simulink model "VIPLStEnCtrl"  (R2018b)
settings: Solver=FixedStepDiscrete  StartTime=0.0  StopTime=10.0  FixedStep=0.01  RelTol=1e-3
undefined symbols (not defined in the file or in its folder): data, DrvStFtEn_Clear, DrvStFtEn_Set, SecRwLtStBkReclnEn_Clear, SecRwLtStBkReclnEn_Set, SecRwLtStFwdBkwdEn_Clear, SecRwLtStFwdBkwdEn_Set, SecRwLtStLgrstUpwdDnwdEn_Clear, SecRwLtStLgrstUpwdDnwdEn_Set, SecRwLtStLtwdRtwdEn_Clear, SecRwLtStLtwdRtwdEn_Set, ThdRwLtStBkReclnEn_Clear, ThdRwLtStBkReclnEn_Set, ThdRwLtStFwdBkwdEn_Clear, ThdRwLtStFwdBkwdEn_Set
libraries: simulink x1
settings Model: Creator=sn2xws  LastModifiedBy=sn2xws
settings DataIOCC: SaveFormat=StructureWithTime
settings OptimizationCC: DefaultParameterBehavior=Inlined  EnhancedBackFolding=on  PassReuseOutputArgsAs=Individual arguments  ZeroExternalMemoryAtStartup=off  ZeroInternalMemoryAtStartup=off  OptimizeBlockOrder=speed  DifferentSizesBufferReuse=on  OptimizationCustomize=off
settings DebuggingCC: ParameterTunabilityLossMsg=error
settings ModelReferenceCC: ModelReferenceNumInstancesAllowed=Single
settings SFSimCC: MATLABDynamicMemAlloc=off
settings RTWCC: SystemTargetFile=autosar.tlc  GenCodeOnly=on  TemplateMakefile=ert_default_tmf  Description=AUTOSAR  GenerateReport=on  IncludeHyperlinkInReport=on  LaunchReport=on  GenerateTraceInfo=on  GenerateTraceReport=on  GenerateTraceReportSl=on  GenerateTraceReportSf=on  GenerateTraceReportEml=on  GenerateCodeMetricsReport=on
settings CodeAppCC: ForceParamTrailComments=on  IgnoreCustomStorageClasses=off  OperatorAnnotations=on  SimulinkDataObjDesc=on  SFDataObjDesc=on  InsertBlockDesc=on
settings STFCustomTargetCC: TargetLangStandard=C99 (ISO)  MultiwordLength=256  ParMdlRefBuildCompliant=on  CompOptLevelCompliant=on  IncludeMdlTerminateFcn=off  CombineOutputUpdateFcns=on  SuppressErrorStatus=on  ERTCustomFileBanners=on  SupportNonFinite=off  SupportComplex=off  SupportContinuousTime=off  SupportNonInlinedSFcns=off  RemoveResetFunc=on  MATLABClassNameForMDSCustomization=Simulink.SoftwareTarget.ERTCustomization  AutosarCompliant=on  UseToolchainInfoCompliant=on  LookupTableObjectStructAxisOrder=2,1,3,4,...  LUTObjectStructOrderEvenSpacing=Size,Table,Breakpoints  SystemTargetFile=autosar.tlc
settings ERTTargetCC: TargetLangStandard=C99 (ISO)  ConcurrentExecutionCompliant=off  IncludeMdlTerminateFcn=off  SuppressErrorStatus=on  SupportNonFinite=off  SupportComplex=off  ModelStepFunctionPrototypeControlCompliant=off  CPPClassGenCompliant=off  AutosarCompliant=on  LookupTableObjectStructAxisOrder=2,1,3,4,...  LUTObjectStructOrderEvenSpacing=Size,Table,Breakpoints  InlinedParameterPlacement=NonHierarchical  ERTCustomFileTemplate=example_file_process.tlc  ERTFilePackagingFormat=Compact

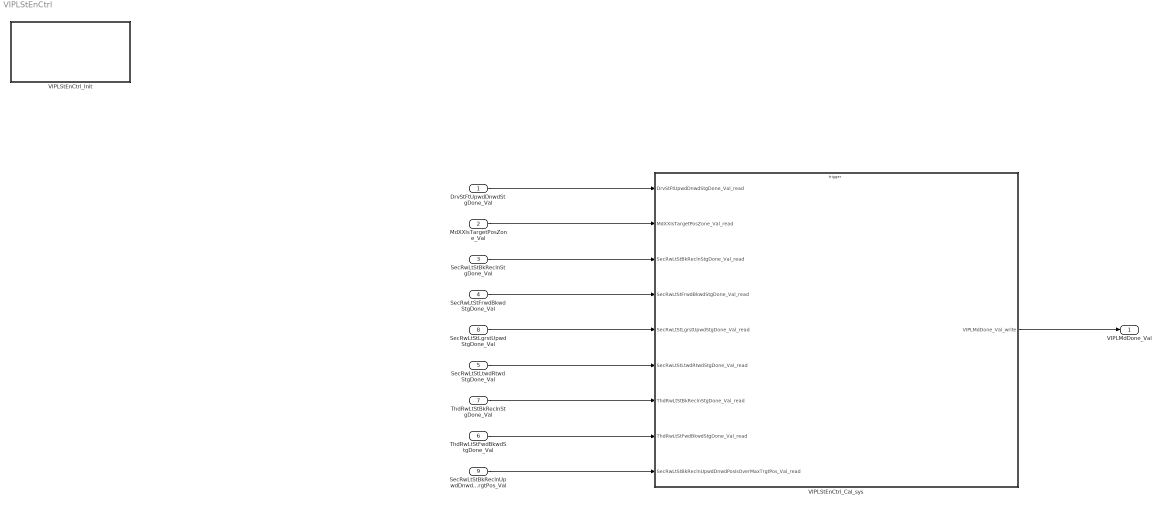
== system VIPLStEnCtrl ==
  DrvStFtUpwdDnwdStgDone_Val : Inport  OutDataTypeStr=boolean  PortDimensions=1
  MdXXIsTargetPosZone_Val : Inport  Port=2  OutDataTypeStr=uint32  PortDimensions=1
  SecRwLtStBkReclnStgDone_Val : Inport  Port=3  OutDataTypeStr=boolean  PortDimensions=1
  SecRwLtStFrwdBkwdStgDone_Val : Inport  Port=4  OutDataTypeStr=boolean  PortDimensions=1
  SecRwLtStLtwdRtwdStgDone_Val : Inport  Port=5  OutDataTypeStr=boolean  PortDimensions=1
  ThdRwLtStFwdBkwdStgDone_Val : Inport  Port=6  OutDataTypeStr=boolean  PortDimensions=1
  ThdRwLtStBkReclnStgDone_Val : Inport  Port=7  OutDataTypeStr=boolean  PortDimensions=1
  SecRwLtStLgrstUpwdStgDone_Val : Inport  Port=8  OutDataTypeStr=boolean  PortDimensions=1
  SecRwLtStBkReclnUpwdDnwdPosIsOverMaxTrgtPos_Val : Inport  Port=9  OutDataTypeStr=boolean  PortDimensions=1
  VIPLStEnCtrl_Cal_sys : Subsystem
  VIPLStEnCtrl_Init : Subsystem
  VIPLMdDone_Val : Outport  OutDataTypeStr=uint8  PortDimensions=1
  wires:
  ThdRwLtStFwdBkwdStgDone_Val/1 -> VIPLStEnCtrl_Cal_sys/8(ThdRwLtStFwdBkwdStgDone_Val_read)
  VIPLStEnCtrl_Cal_sys/1(VIPLMdDone_Val_write) -> VIPLMdDone_Val/1
  DrvStFtUpwdDnwdStgDone_Val/1 -> VIPLStEnCtrl_Cal_sys/1(DrvStFtUpwdDnwdStgDone_Val_read)
  MdXXIsTargetPosZone_Val/1 -> VIPLStEnCtrl_Cal_sys/2(MdXXIsTargetPosZone_Val_read)
  SecRwLtStBkReclnStgDone_Val/1 -> VIPLStEnCtrl_Cal_sys/3(SecRwLtStBkReclnStgDone_Val_read)
  SecRwLtStFrwdBkwdStgDone_Val/1 -> VIPLStEnCtrl_Cal_sys/4(SecRwLtStFrwdBkwdStgDone_Val_read)
  SecRwLtStLgrstUpwdStgDone_Val/1 -> VIPLStEnCtrl_Cal_sys/5(SecRwLtStLgrstUpwdStgDone_Val_read)
  SecRwLtStLtwdRtwdStgDone_Val/1 -> VIPLStEnCtrl_Cal_sys/6(SecRwLtStLtwdRtwdStgDone_Val_read)
  ThdRwLtStBkReclnStgDone_Val/1 -> VIPLStEnCtrl_Cal_sys/7(ThdRwLtStBkReclnStgDone_Val_read)
  SecRwLtStBkReclnUpwdDnwdPosIsOverMaxTrgtPos_Val/1 -> VIPLStEnCtrl_Cal_sys/9(SecRwLtStBkReclnUpwdDnwdPosIsOverMaxTrgtPos_Val_read)

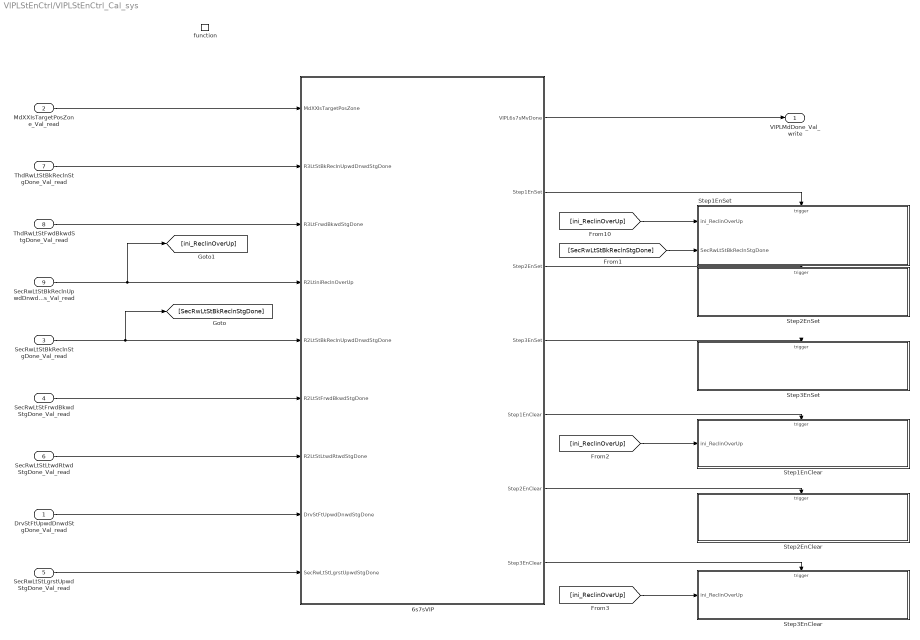
== system VIPLStEnCtrl/VIPLStEnCtrl_Cal_sys ==
  DrvStFtUpwdDnwdStgDone_Val_read : Inport
  MdXXIsTargetPosZone_Val_read : Inport  Port=2
  SecRwLtStBkReclnStgDone_Val_read : Inport  Port=3
  SecRwLtStFrwdBkwdStgDone_Val_read : Inport  Port=4
  SecRwLtStLgrstUpwdStgDone_Val_read : Inport  Port=5
  SecRwLtStLtwdRtwdStgDone_Val_read : Inport  Port=6
  ThdRwLtStBkReclnStgDone_Val_read : Inport  Port=7
  ThdRwLtStFwdBkwdStgDone_Val_read : Inport  Port=8
  SecRwLtStBkReclnUpwdDnwdPosIsOverMaxTrgtPos_Val_read : Inport  Port=9
  function : TriggerPort  TriggerType=function-call  IsSimulinkFunction=on  FunctionName=VIPLStEnCtrl_Cal  VariantControl=(inherit)
  6s7sVIP : Subsystem
  Step1EnClear : Subsystem  TreatAsAtomicUnit=on
  Step1EnSet : Subsystem  TreatAsAtomicUnit=on
  Step2EnClear : Subsystem  TreatAsAtomicUnit=on
  Step2EnSet : Subsystem  TreatAsAtomicUnit=on
  Step3EnClear : Subsystem  TreatAsAtomicUnit=on
  Step3EnSet : Subsystem  TreatAsAtomicUnit=on
  VIPLMdDone_Val_write : Outport
      settings: EnsureOutportIsVirtual=on
  wires:
  6s7sVIP/1(VIPL6s7sMvDone) -> VIPLMdDone_Val_write/1
  MdXXIsTargetPosZone_Val_read/1 -> 6s7sVIP/1(MdXXIsTargetPosZone)
  ThdRwLtStBkReclnStgDone_Val_read/1 -> 6s7sVIP/2(R3LtStBkReclnUpwdDnwdStgDone)
  ThdRwLtStFwdBkwdStgDone_Val_read/1 -> 6s7sVIP/3(R3LtFrwdBkwdStgDone)
  SecRwLtStBkReclnStgDone_Val_read/1 -> [SecRwLtStBkReclnStgDone], 6s7sVIP/5(R2LtStBkReclnUpwdDnwdStgDone)
  SecRwLtStFrwdBkwdStgDone_Val_read/1 -> 6s7sVIP/6(R2LtStFrwdBkwdStgDone)
  SecRwLtStLtwdRtwdStgDone_Val_read/1 -> 6s7sVIP/7(R2LtStLtwdRtwdStgDone)
  SecRwLtStLgrstUpwdStgDone_Val_read/1 -> 6s7sVIP/9(SecRwLtStLgrstUpwdStgDone)
  DrvStFtUpwdDnwdStgDone_Val_read/1 -> 6s7sVIP/8(DrvStFtUpwdDnwdStgDone)
  [ini_ReclinOverUp] -> Step1EnSet/1(ini_ReclinOverUp)
  6s7sVIP/6(Step2EnClear) -> Step2EnClear/Trigger
  6s7sVIP/7(Step3EnClear) -> Step3EnClear/Trigger
  6s7sVIP/4(Step3EnSet) -> Step3EnSet/Trigger
  [SecRwLtStBkReclnStgDone] -> Step1EnSet/2(SecRwLtStBkReclnStgDone)
  6s7sVIP/3(Step2EnSet) -> Step2EnSet/Trigger
  6s7sVIP/2(Step1EnSet) -> Step1EnSet/Trigger
  6s7sVIP/5(Step1EnClear) -> Step1EnClear/Trigger
  [ini_ReclinOverUp] -> Step1EnClear/1(ini_ReclinOverUp)
  [ini_ReclinOverUp] -> Step3EnClear/1(ini_ReclinOverUp)
  SecRwLtStBkReclnUpwdDnwdPosIsOverMaxTrgtPos_Val_read/1 -> [ini_ReclinOverUp], 6s7sVIP/4(R2LtiniReclnOverUp)

== system VIPLStEnCtrl/VIPLStEnCtrl_Init ==
  Event Listener : EventListener  EventName=reset

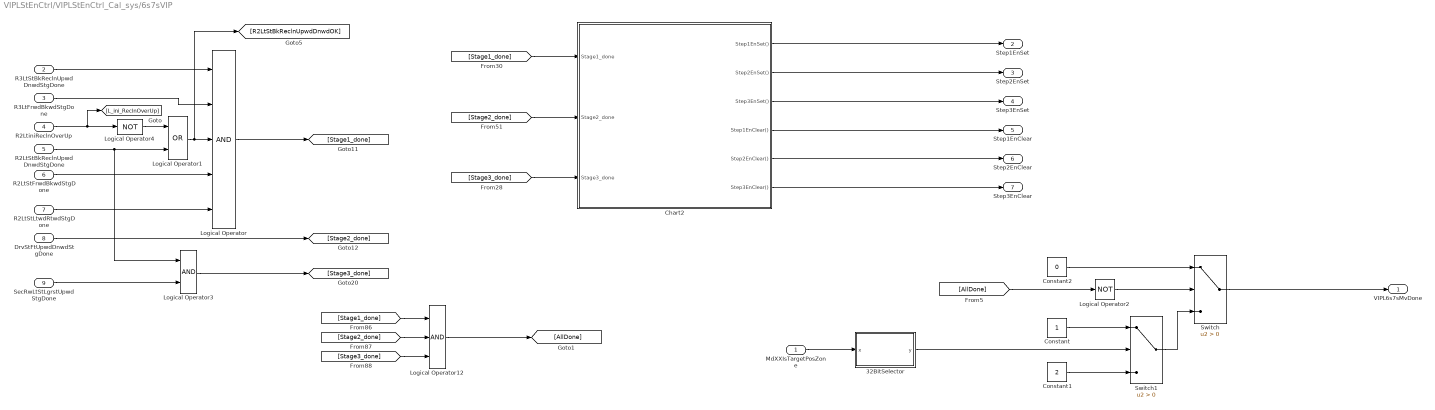
== system VIPLStEnCtrl/VIPLStEnCtrl_Cal_sys/6s7sVIP ==
  MdXXIsTargetPosZone : Inport
  R3LtStBkReclnUpwdDnwdStgDone : Inport  Port=2
  R3LtFrwdBkwdStgDone : Inport  Port=3
  R2LtiniReclnOverUp : Inport  Port=4
  R2LtStBkReclnUpwdDnwdStgDone : Inport  Port=5
  R2LtStFrwdBkwdStgDone : Inport  Port=6
  R2LtStLtwdRtwdStgDone : Inport  Port=7
  DrvStFtUpwdDnwdStgDone : Inport  Port=8
  SecRwLtStLgrstUpwdStgDone : Inport  Port=9
  32BitSelector : Subsystem  mask(32 Bit Selector){BitNum=9}
      mask prompts: BitNum "Select Bit Number"
      mask help: Allows selection of a particular bit (0-31) out of a packed word up to 32 bits long. Output will be true if the bit number selected via the mask parameter is equal to one.
      mask TypeOptions BitNum: 0 | 1 | 2 | 3 | 4 | 5 | 6 | 7 | 8 | 9 | 10 | 11 | 12 | 13 | 14 | 15 | 16 | 17 | 18 | 19 | 20 | 21 | 22 | 23 | 24 | 25 | 26 | 27 | 28 | 29 | 30 | 31
      mask Display:
      | text(0.5, 0.8,'BIT','horizontalAlignment','center')
      | text(0.5, 0.5,'SELECTOR','horizontalAlignment','center')
      | text(0.5, 0.2,['-- Bit ',char(get_param(gcb,'BitNum')),' --'],'horizontalAlignment','center')
  Chart2 : Stateflow chart  TreatAsAtomicUnit=on
  Constant : Constant  OutDataTypeStr=uint8
  Constant1 : Constant  Value=2  OutDataTypeStr=uint8
  Constant2 : Constant  Value=0  OutDataTypeStr=uint8
  Logical Operator : Logic  Inputs=5  AllPortsSameDT=off  OutDataTypeStr=boolean
  Logical Operator1 : Logic  Operator=OR  AllPortsSameDT=off  OutDataTypeStr=boolean
  Logical Operator12 : Logic  Inputs=3  AllPortsSameDT=off  OutDataTypeStr=boolean
  Logical Operator2 : Logic  Operator=NOT  AllPortsSameDT=off  OutDataTypeStr=boolean
  Logical Operator3 : Logic  AllPortsSameDT=off  OutDataTypeStr=boolean
  Logical Operator4 : Logic  Operator=NOT  AllPortsSameDT=off  OutDataTypeStr=boolean
  Switch : Switch  Criteria=u2 > Threshold
  Switch1 : Switch  Criteria=u2 > Threshold
  VIPL6s7sMvDone : Outport
  Step1EnSet : Outport  Port=2
  Step2EnSet : Outport  Port=3
  Step3EnSet : Outport  Port=4
  Step1EnClear : Outport  Port=5
  Step2EnClear : Outport  Port=6
  Step3EnClear : Outport  Port=7
  wires:
  [Stage1_done] -> Chart2/1(Stage1_done)
  SecRwLtStLgrstUpwdStgDone/1 -> Logical Operator3/2
  Logical Operator4/1 -> Logical Operator1/1
  [Stage3_done] -> Logical Operator12/3
  R3LtFrwdBkwdStgDone/1 -> Logical Operator/2
  [Stage2_done] -> Chart2/2(Stage2_done)
  R2LtStBkReclnUpwdDnwdStgDone/1 -> Logical Operator1/2, Logical Operator3/1
  Logical Operator1/1 -> [R2LtStBkReclnUpwdDnwdOK], Logical Operator/3
  Logical Operator/1 -> [Stage1_done]
  R3LtStBkReclnUpwdDnwdStgDone/1 -> Logical Operator/1
  Logical Operator3/1 -> [Stage3_done]
  R2LtiniReclnOverUp/1 -> [L_ini_ReclnOverUp], Logical Operator4/1
  R2LtStFrwdBkwdStgDone/1 -> Logical Operator/4
  DrvStFtUpwdDnwdStgDone/1 -> [Stage2_done]
  MdXXIsTargetPosZone/1 -> 32BitSelector/1(x)
  Logical Operator12/1 -> [AllDone]
  [Stage2_done] -> Logical Operator12/2
  R2LtStLtwdRtwdStgDone/1 -> Logical Operator/5
  [Stage1_done] -> Logical Operator12/1
  [Stage3_done] -> Chart2/3(Stage3_done)
  Chart2/1(Step1EnSet()) -> Step1EnSet/1
  Chart2/2(Step2EnSet()) -> Step2EnSet/1
  Chart2/3(Step3EnSet()) -> Step3EnSet/1
  Chart2/4(Step1EnClear()) -> Step1EnClear/1
  Chart2/5(Step2EnClear()) -> Step2EnClear/1
  Chart2/6(Step3EnClear()) -> Step3EnClear/1
  Switch1/1 -> Switch/3
  Switch/1 -> VIPL6s7sMvDone/1
  Constant2/1 -> Switch/1
  Constant1/1 -> Switch1/3
  Constant/1 -> Switch1/1
  Logical Operator2/1 -> Switch/2
  [AllDone] -> Logical Operator2/1
  32BitSelector/1(y) -> Switch1/2

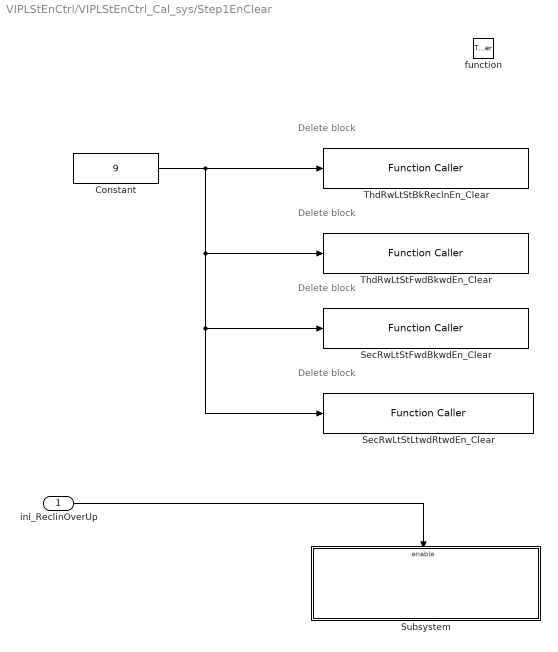
== system VIPLStEnCtrl/VIPLStEnCtrl_Cal_sys/Step1EnClear ==
  note: Delete block
  note: Delete block
  note: Delete block
  note: Delete block
  ini_ReclinOverUp : Inport
  function : TriggerPort  TriggerType=function-call  VariantControl=Variant
  Constant : Constant  Value=9  OutDataTypeStr=uint8
  SecRwLtStFwdBkwdEn_Clear : FunctionCaller  FunctionPrototype=SecRwLtStFwdBkwdEn_Clear(data)  InputArgumentSpecifications=uint8(1)
  SecRwLtStLtwdRtwdEn_Clear : FunctionCaller  FunctionPrototype=SecRwLtStLtwdRtwdEn_Clear(data)  InputArgumentSpecifications=uint8(1)
  Subsystem : Subsystem
  ThdRwLtStBkReclnEn_Clear : FunctionCaller  FunctionPrototype=ThdRwLtStBkReclnEn_Clear(data)  InputArgumentSpecifications=uint8(1)
  ThdRwLtStFwdBkwdEn_Clear : FunctionCaller  FunctionPrototype=ThdRwLtStFwdBkwdEn_Clear(data)  InputArgumentSpecifications=uint8(1)
  wires:
  Constant/1 -> ThdRwLtStBkReclnEn_Clear/1, SecRwLtStFwdBkwdEn_Clear/1, SecRwLtStLtwdRtwdEn_Clear/1, ThdRwLtStFwdBkwdEn_Clear/1
  ini_ReclinOverUp/1 -> Subsystem/Enable

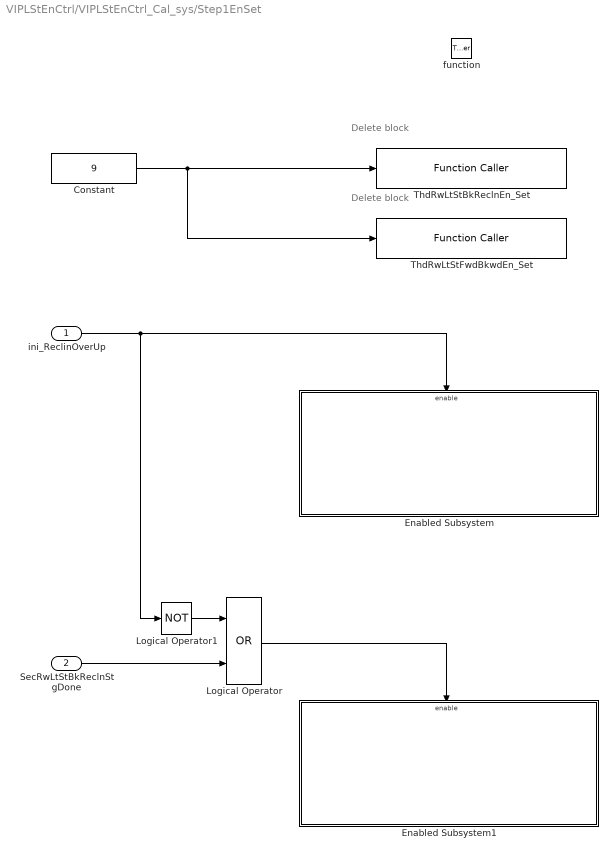
== system VIPLStEnCtrl/VIPLStEnCtrl_Cal_sys/Step1EnSet ==
  note: Delete block
  note: Delete block
  ini_ReclinOverUp : Inport
  SecRwLtStBkReclnStgDone : Inport  Port=2
  function : TriggerPort  TriggerType=function-call  VariantControl=Variant
  Constant : Constant  Value=9  OutDataTypeStr=uint8
  Enabled Subsystem : Subsystem  TreatAsAtomicUnit=on
  Enabled Subsystem1 : Subsystem  TreatAsAtomicUnit=on
  Logical Operator : Logic  Operator=OR  AllPortsSameDT=off  OutDataTypeStr=boolean
  Logical Operator1 : Logic  Operator=NOT  AllPortsSameDT=off  OutDataTypeStr=boolean
  ThdRwLtStBkReclnEn_Set : FunctionCaller  FunctionPrototype=ThdRwLtStBkReclnEn_Set(data)  InputArgumentSpecifications=uint8(1)
  ThdRwLtStFwdBkwdEn_Set : FunctionCaller  FunctionPrototype=ThdRwLtStFwdBkwdEn_Set(data)  InputArgumentSpecifications=uint8(1)
  wires:
  Constant/1 -> ThdRwLtStBkReclnEn_Set/1, ThdRwLtStFwdBkwdEn_Set/1
  ini_ReclinOverUp/1 -> Logical Operator1/1, Enabled Subsystem/Enable
  SecRwLtStBkReclnStgDone/1 -> Logical Operator/2
  Logical Operator1/1 -> Logical Operator/1
  Logical Operator/1 -> Enabled Subsystem1/Enable

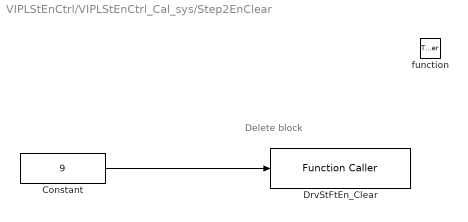
== system VIPLStEnCtrl/VIPLStEnCtrl_Cal_sys/Step2EnClear ==
  note: Delete block
  function : TriggerPort  TriggerType=function-call  VariantControl=Variant
  Constant : Constant  Value=9  OutDataTypeStr=uint8
  DrvStFtEn_Clear : FunctionCaller  FunctionPrototype=DrvStFtEn_Clear(data)  InputArgumentSpecifications=uint8(1)
  wires:
  Constant/1 -> DrvStFtEn_Clear/1

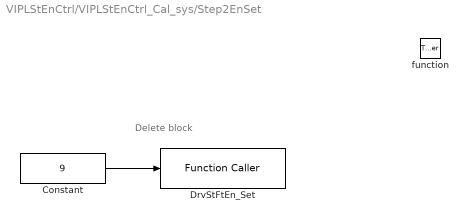
== system VIPLStEnCtrl/VIPLStEnCtrl_Cal_sys/Step2EnSet ==
  note: Delete block
  function : TriggerPort  TriggerType=function-call  VariantControl=Variant
  Constant : Constant  Value=9  OutDataTypeStr=uint8
  DrvStFtEn_Set : FunctionCaller  FunctionPrototype=DrvStFtEn_Set(data)  InputArgumentSpecifications=uint8(1)
  wires:
  Constant/1 -> DrvStFtEn_Set/1

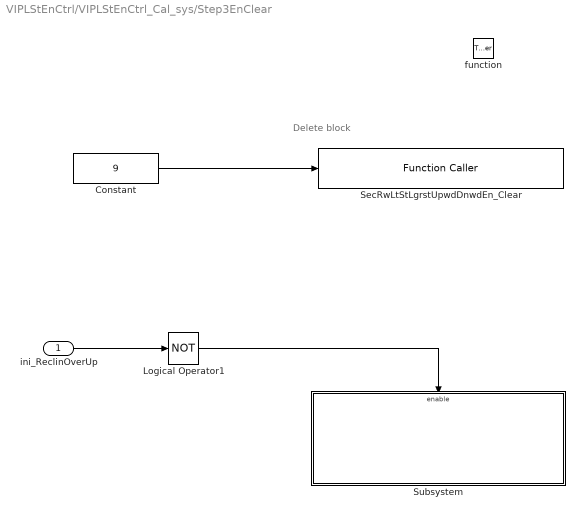
== system VIPLStEnCtrl/VIPLStEnCtrl_Cal_sys/Step3EnClear ==
  note: Delete block
  ini_ReclinOverUp : Inport
  function : TriggerPort  TriggerType=function-call  VariantControl=Variant
  Constant : Constant  Value=9  OutDataTypeStr=uint8
  Logical Operator1 : Logic  Operator=NOT  AllPortsSameDT=off  OutDataTypeStr=boolean
  SecRwLtStLgrstUpwdDnwdEn_Clear : FunctionCaller  FunctionPrototype=SecRwLtStLgrstUpwdDnwdEn_Clear(data)  InputArgumentSpecifications=uint8(1)
  Subsystem : Subsystem
  wires:
  Constant/1 -> SecRwLtStLgrstUpwdDnwdEn_Clear/1
  ini_ReclinOverUp/1 -> Logical Operator1/1
  Logical Operator1/1 -> Subsystem/Enable

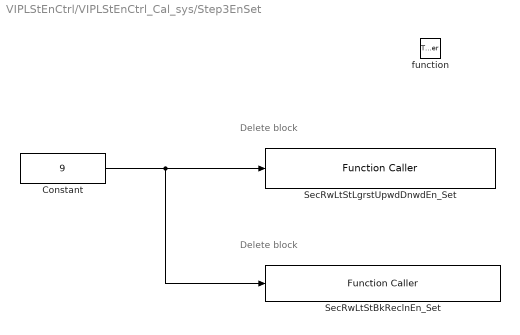
== system VIPLStEnCtrl/VIPLStEnCtrl_Cal_sys/Step3EnSet ==
  note: Delete block
  note: Delete block
  function : TriggerPort  TriggerType=function-call  VariantControl=Variant
  Constant : Constant  Value=9  OutDataTypeStr=uint8
  SecRwLtStBkReclnEn_Set : FunctionCaller  FunctionPrototype=SecRwLtStBkReclnEn_Set(data)  InputArgumentSpecifications=uint8(1)
  SecRwLtStLgrstUpwdDnwdEn_Set : FunctionCaller  FunctionPrototype=SecRwLtStLgrstUpwdDnwdEn_Set(data)  InputArgumentSpecifications=uint8(1)
  wires:
  Constant/1 -> SecRwLtStBkReclnEn_Set/1, SecRwLtStLgrstUpwdDnwdEn_Set/1

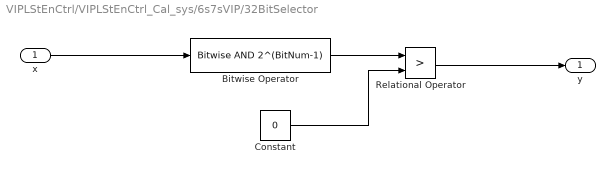
== system VIPLStEnCtrl/VIPLStEnCtrl_Cal_sys/6s7sVIP/32BitSelector ==
  x : Inport
  Bitwise Operator : simulink/Logic and Bit Operations/Bitwise Operator  logicop=AND  UseBitMask=on  BitMask=2^(BitNum-1)  BitMaskRealWorld=Stored Integer
  Constant : Constant  Value=0  OutDataTypeStr=uint32
  Relational Operator : RelationalOperator  Operator=>  OutDataTypeStr=boolean  RndMeth=Simplest
  y : Outport
  wires:
  Relational Operator/1 -> y/1
  Constant/1 -> Relational Operator/2
  x/1 -> Bitwise Operator/1
  Bitwise Operator/1 -> Relational Operator/1

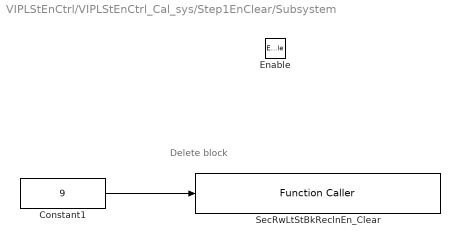
== system VIPLStEnCtrl/VIPLStEnCtrl_Cal_sys/Step1EnClear/Subsystem ==
  note: Delete block
  Enable : EnablePort
  Constant1 : Constant  Value=9  OutDataTypeStr=uint8
  SecRwLtStBkReclnEn_Clear : FunctionCaller  FunctionPrototype=SecRwLtStBkReclnEn_Clear(data)  InputArgumentSpecifications=uint8(1)
  wires:
  Constant1/1 -> SecRwLtStBkReclnEn_Clear/1

== system VIPLStEnCtrl/VIPLStEnCtrl_Cal_sys/Step1EnSet/Enabled Subsystem ==
  note: Delete block
  Enable : EnablePort
  Constant : Constant  Value=9  OutDataTypeStr=uint8
  SecRwLtStBkReclnEn_Set : FunctionCaller  FunctionPrototype=SecRwLtStBkReclnEn_Set(data)  InputArgumentSpecifications=uint8(1)
  wires:
  Constant/1 -> SecRwLtStBkReclnEn_Set/1

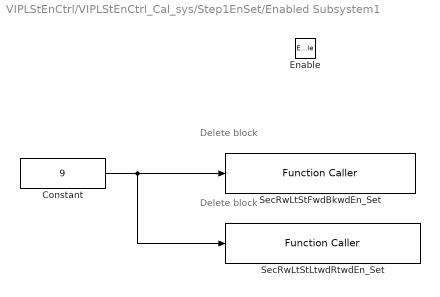
== system VIPLStEnCtrl/VIPLStEnCtrl_Cal_sys/Step1EnSet/Enabled Subsystem1 ==
  note: Delete block
  note: Delete block
  Enable : EnablePort
  Constant : Constant  Value=9  OutDataTypeStr=uint8
  SecRwLtStFwdBkwdEn_Set : FunctionCaller  FunctionPrototype=SecRwLtStFwdBkwdEn_Set(data)  InputArgumentSpecifications=uint8(1)
  SecRwLtStLtwdRtwdEn_Set : FunctionCaller  FunctionPrototype=SecRwLtStLtwdRtwdEn_Set(data)  InputArgumentSpecifications=uint8(1)
  wires:
  Constant/1 -> SecRwLtStFwdBkwdEn_Set/1, SecRwLtStLtwdRtwdEn_Set/1

== system VIPLStEnCtrl/VIPLStEnCtrl_Cal_sys/Step3EnClear/Subsystem ==
  note: Delete block
  Enable : EnablePort
  Constant1 : Constant  Value=9  OutDataTypeStr=uint8
  SecRwLtStBkReclnEn_Clear : FunctionCaller  FunctionPrototype=SecRwLtStBkReclnEn_Clear(data)  InputArgumentSpecifications=uint8(1)
  wires:
  Constant1/1 -> SecRwLtStBkReclnEn_Clear/1

== stateflow chart VIPLStEnCtrl/VIPLStEnCtrl_Cal_sys/6s7sVIP/Chart2 ==
  (default) -> (junction 616)
  (junction 616) -> (junction 618) [order 1] : [!Stage1_done]
  (junction 616) -> (junction 622) [order 2]
  (junction 618) -> (junction 620) : {
      | Step1EnSet;
      | Step2EnClear;
      | Step3EnClear;
      | }
  (junction 622) -> (junction 624) [order 1] : [!Stage2_done]
  (junction 622) -> (junction 629) [order 2]
  (junction 624) -> (junction 626) : {
      | Step1EnClear;
      | Step2EnSet;
      | Step3EnClear;
      | }
  (junction 629) -> (junction 631) [order 1] : [!Stage3_done]
  (junction 629) -> (junction 636) [order 2] : {
      | Step1EnClear;
      | Step2EnClear;
      | Step3EnClear;
      | }
  (junction 631) -> (junction 633) : {
      | Step1EnClear;
      | Step2EnClear;
      | Step3EnSet;
      | }
  (junction 633) -> (junction 636)
  (junction 626) -> (junction 633)
  (junction 620) -> (junction 626)
  (junction 636) -> (junction 639)
  data: Stage1_done input boolean; Stage2_done input boolean; Stage3_done input boolean
  events: Step1EnSet output FUNCTION_CALL_EVENT; Step2EnSet output FUNCTION_CALL_EVENT; Step3EnSet output FUNCTION_CALL_EVENT; Step1EnClear output FUNCTION_CALL_EVENT; Step2EnClear output FUNCTION_CALL_EVENT; Step3EnClear output FUNCTION_CALL_EVENT
